simulink model "simulink_model_1"  (R2021b)
settings: Solver=VariableStepAuto  StartTime=0.0  StopTime=50.0  RelTol=1e-3
settings Model: Creator=Admin  LastModifiedBy=Admin

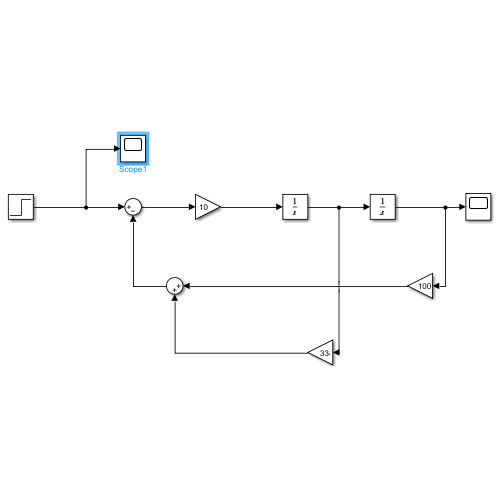
[thumbnail: Simulink's stored preview of the top-level diagram]
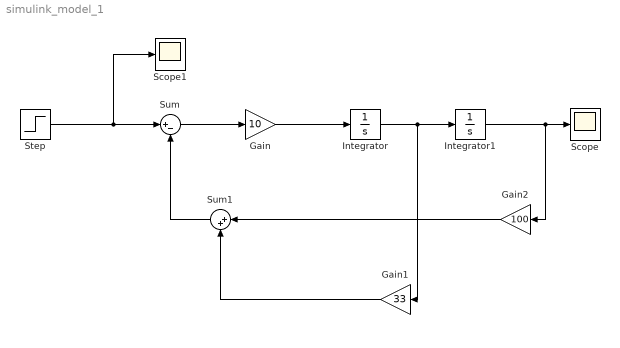
== system simulink_model_1 ==
  Gain : Gain  Gain=10
  Gain1 : Gain  Gain=33
  Gain2 : Gain  Gain=100
  Integrator : Integrator
  Integrator1 : Integrator
  Scope : Scope
  Scope1 : Scope
  Step : Step  Time=10  SampleTime=0
  Sum : Sum  Inputs=|+-
  Sum1 : Sum  Inputs=|++
  wires:
  Sum/1 -> Gain/1
  Step/1 -> Scope1/1, Sum/1
  Sum1/1 -> Sum/2
  Integrator/1 -> Gain1/1, Integrator1/1
  Integrator1/1 -> Gain2/1, Scope/1
  Gain/1 -> Integrator/1
  Gain1/1 -> Sum1/2
  Gain2/1 -> Sum1/1
